simulink model "circuit7R"  (Simulink 5.0)
settings: Solver=ode45  StartTime=0.0  StopTime=0.1  RelTol=1e-3
libraries: powerlib2 x9, simulink x1
settings Model: LastModifiedBy=pavel  SimulationMode=accelerator

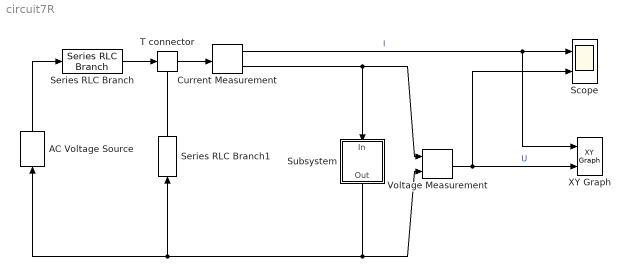
== system circuit7R ==
  AC Voltage Source : powerlib2/Electrical Sources/AC Voltage Source  Tag=PoWeRsYsTeMbLoCk  Description=source block  Orientation=up  A=120e3/sqrt(3)*sqrt(2)*2.3  P=0  F=60  stime=0  mesure=None  PSBOutputType=1
  Current Measurement : powerlib2/Measurements/Current Measurement  Tag=PoWeRsYsTeMmEaSuReMeNt  PhasorSimulation=off  OutputType=Magnitude  PSBOutputType=01  PSBequivalent=0
  Scope : Scope  NumInputPorts=2
      settings: YMin=-1750~-2e+007  YMax=1750~2.25e+007
  Series RLC Branch : powerlib2/Elements/Series RLC Branch  Tag=PoWeRsYsTeMbLoCk  a=1.92  b=26e-3  c=inf  mesure=None  PSBOutputType=1
  Series RLC Branch1 : powerlib2/Elements/Series RLC Branch  Tag=PoWeRsYsTeMbLoCk  Orientation=up  a=10e6  b=0  c=inf  mesure=None  PSBOutputType=1
  Subsystem : Subsystem  Orientation=down  mask(Nonlinear Inductance){Vo=120e3/sqrt(3)*sqrt(2)*2, Io=500, alpha=25}
      mask prompts: Vo "Protect voltage"; Io "Reference current"
  T connector : powerlib2/Connectors/T connector  Tag=PoWeRsYsTeMbLoCk  PSBOutputType=1
  Voltage Measurement : powerlib2/Measurements/Voltage Measurement  Tag=PoWeRsYsTeMmEaSuReMeNt  PhasorSimulation=off  OutputType=Magnitude  PSBOutputType=0  PSBequivalent=1
  XY Graph : simulink/Sinks/XY Graph  xmin=-2000  xmax=2000  ymin=-2.5e5  ymax=2.5e5  st=-1
  wires:
  AC Voltage Source/1 -> Series RLC Branch/1
  Series RLC Branch/1 -> T connector/1
  Current Measurement/2 -> Subsystem/1(In), Voltage Measurement/1
  Subsystem/1(Out) -> AC Voltage Source/1, Series RLC Branch1/1, Voltage Measurement/2
  T connector/1 -> Current Measurement/1
  Series RLC Branch1/1 -> T connector/Enable
  Current Measurement/1 -> Scope/1, XY Graph/1  "I"
  Voltage Measurement/1 -> Scope/2, XY Graph/2  "U"

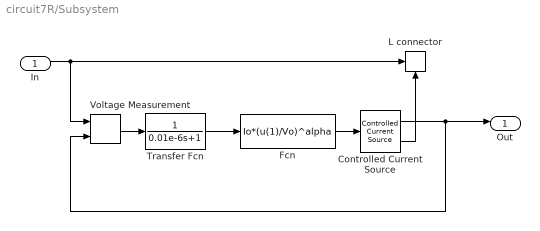
== system circuit7R/Subsystem ==
  In : Inport
  Controlled Current Source : powerlib2/Electrical Sources/Controlled Current Source  Tag=PoWeRsYsTeMbLoCk  Description=source block  initsrc=on  srctyp=AC  ia=0  iph=0  freq=0  mesure=None  PSBOutputType=11
  Fcn : Fcn  Expr=Io*(u(1)/Vo)^alpha
  L connector : powerlib2/Connectors/L connector  Tag=PoWeRsYsTeMbLoCk  Orientation=up
  Transfer Fcn : TransferFcn  Denominator=[0.01e-6 1]
  Voltage Measurement : powerlib2/Measurements/Voltage Measurement  Tag=PoWeRsYsTeMmEaSuReMeNt  PhasorSimulation=off  OutputType=Magnitude  PSBOutputType=0  PSBequivalent=0
  Out : Outport
  wires:
  Voltage Measurement/1 -> Transfer Fcn/1
  In/1 -> L connector/Enable, Voltage Measurement/1
  Controlled Current Source/2 -> L connector/1
  Controlled Current Source/1 -> Voltage Measurement/2, Out/1
  Fcn/1 -> Controlled Current Source/1
  Transfer Fcn/1 -> Fcn/1
